simulink model "lab1"  (R2018b)
settings: Solver=FixedStepAuto  StartTime=0.0  StopTime=10.0  FixedStep=.001  RelTol=1e-3
undefined symbols (not defined in the file or in its folder): J, K1, K2, Komg, Kv, M
libraries: simulink x1
settings Model: Creator=FetCatz  LastModifiedBy=FetCatz
settings SolverCC: ZeroCrossControl=DisableAll  AutoInsertRateTranBlk=on

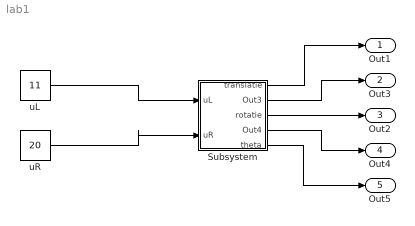
== system lab1 ==
  Subsystem : Subsystem
  uL : Constant  Value=11
  uR : Constant  Value=20
  Out1 : Outport
  Out3 : Outport  Port=2
  Out2 : Outport  Port=3
  Out4 : Outport  Port=4
  Out5 : Outport  Port=5
  wires:
  Subsystem/1(translatie) -> Out1/1
  Subsystem/2(Out3) -> Out3/1
  Subsystem/3(rotatie) -> Out2/1
  Subsystem/4(Out4) -> Out4/1
  Subsystem/5(theta) -> Out5/1
  uR/1 -> Subsystem/2(uR)
  uL/1 -> Subsystem/1(uL)

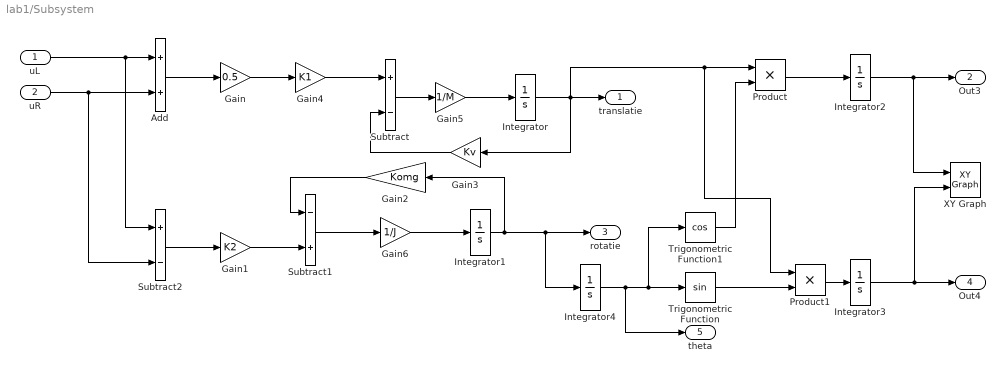
== system lab1/Subsystem ==
  uL : Inport
  uR : Inport  Port=2
  Add : Sum
  Gain : Gain  Gain=0.5
  Gain1 : Gain  Gain=K2
  Gain2 : Gain  Gain=Komg
  Gain3 : Gain  Gain=Kv
  Gain4 : Gain  Gain=K1
  Gain5 : Gain  Gain=1/M
  Gain6 : Gain  Gain=1/J
  Integrator{,1..4} (5 alike) : Integrator
  Product : Product
  Product1 : Product
  Subtract : Sum  Inputs=+-
  Subtract1 : Sum  Inputs=-+
  Subtract2 : Sum  Inputs=+-
  Trigonometric Function : Trigonometry
  Trigonometric Function1 : Trigonometry  Operator=cos
  XY Graph : simulink/Sinks/XY Graph  xmin=-.1  xmax=.1  ymin=-.1  ymax=.1  st=-1
  translatie : Outport
  Out3 : Outport  Port=2
  rotatie : Outport  Port=3
  Out4 : Outport  Port=4
  theta : Outport  Port=5
  wires:
  Integrator2/1 -> XY Graph/1, Out3/1
  Integrator3/1 -> XY Graph/2, Out4/1
  Trigonometric Function/1 -> Product1/2
  uL/1 -> Subtract2/1, Add/1
  Subtract/1 -> Gain5/1
  Gain/1 -> Gain4/1
  Gain4/1 -> Subtract/1
  Product1/1 -> Integrator3/1
  Integrator/1 -> translatie/1, Gain3/1, Product1/1, Product/1
  Gain5/1 -> Integrator/1
  Gain3/1 -> Subtract/2
  Integrator1/1 -> Gain2/1, rotatie/1, Integrator4/1
  uR/1 -> Subtract2/2, Add/2
  Add/1 -> Gain/1
  Gain6/1 -> Integrator1/1
  Gain1/1 -> Subtract1/2
  Gain2/1 -> Subtract1/1
  Trigonometric Function1/1 -> Product/2
  Subtract2/1 -> Gain1/1
  Integrator4/1 -> theta/1, Trigonometric Function/1, Trigonometric Function1/1
  Product/1 -> Integrator2/1
  Subtract1/1 -> Gain6/1
